simulink library "threeTethers_cl"  (R2018b)
settings: Solver=VariableStepAuto  StartTime=0.0  StopTime=10.0  RelTol=1e-3
undefined symbols (not defined in the file): grav, initEulerAngles, initPos, rho, rho_tether, rotation_sequence, sim_param, thr1Pt, thr2Pt, thr3Pt
libraries: singleTether_cl x3
settings Model: Creator=mcobb  LastModifiedBy=Erin B

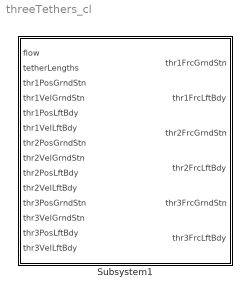
== system threeTethers_cl ==
  Subsystem1 : Subsystem

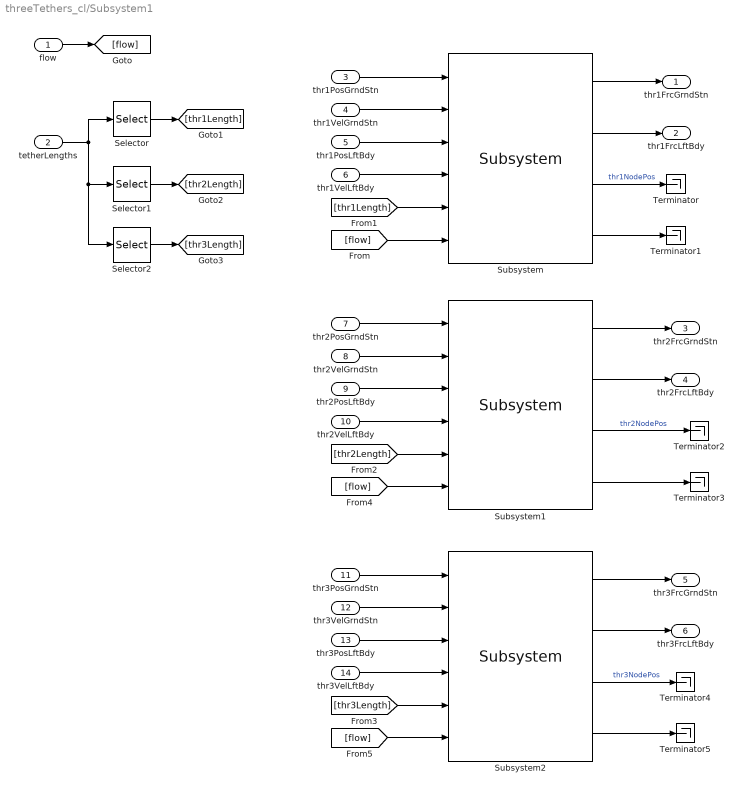
== system threeTethers_cl/Subsystem1 ==
  flow : Inport
  tetherLengths : Inport  Port=2
  thr1PosGrndStn : Inport  Port=3
  thr1VelGrndStn : Inport  Port=4
  thr1PosLftBdy : Inport  Port=5
  thr1VelLftBdy : Inport  Port=6
  thr2PosGrndStn : Inport  Port=7
  thr2VelGrndStn : Inport  Port=8
  thr2PosLftBdy : Inport  Port=9
  thr2VelLftBdy : Inport  Port=10
  thr3PosGrndStn : Inport  Port=11
  thr3VelGrndStn : Inport  Port=12
  thr3PosLftBdy : Inport  Port=13
  thr3VelLftBdy : Inport  Port=14
  Selector : Selector  InputPortWidth=3  IndexOptions=Index vector (dialog)  Indices=1  OutputSizes=1
  Selector1 : Selector  InputPortWidth=3  IndexOptions=Index vector (dialog)  Indices=2  OutputSizes=1
  Selector2 : Selector  InputPortWidth=3  IndexOptions=Index vector (dialog)  Indices=3  OutputSizes=1
  Subsystem : singleTether_cl/Subsystem  N=sim_param.N  dia_t=dia_t  E=E  rho_tether=rho + rho_tether  Cd=Cd  zeta=zeta  rho=rho  g=grav  mass=mass  ini_Rn_o=initPos + (rotation_sequence(initEulerAngles)*thr1Pt')'  ini_R1_o=thr1GndPos
  Subsystem1 : singleTether_cl/Subsystem  N=sim_param.N  dia_t=dia_t  E=E  rho_tether=rho + rho_tether  Cd=Cd  zeta=zeta  rho=rho  g=grav  mass=mass  ini_Rn_o=initPos + (rotation_sequence(initEulerAngles)*thr2Pt')'  ini_R1_o=thr2GndPos
  Subsystem2 : singleTether_cl/Subsystem  N=sim_param.N  dia_t=dia_t  E=E  rho_tether=rho + rho_tether  Cd=Cd  zeta=zeta  rho=rho  g=grav  mass=mass  ini_Rn_o=initPos + (rotation_sequence(initEulerAngles)*thr3Pt')'  ini_R1_o=thr3GndPos
  Terminator{,1..5} (6 alike) : Terminator
  thr1FrcGrndStn : Outport
  thr1FrcLftBdy : Outport  Port=2
  thr2FrcGrndStn : Outport  Port=3
  thr2FrcLftBdy : Outport  Port=4
  thr3FrcGrndStn : Outport  Port=5
  thr3FrcLftBdy : Outport  Port=6
  wires:
  thr1PosGrndStn/1 -> Subsystem/1
  thr1VelGrndStn/1 -> Subsystem/2
  thr1VelLftBdy/1 -> Subsystem/4
  thr1PosLftBdy/1 -> Subsystem/3
  flow/1 -> [flow]
  [flow] -> Subsystem/6
  Selector/1 -> [thr1Length]
  tetherLengths/1 -> Selector/1, Selector1/1, Selector2/1
  Selector1/1 -> [thr2Length]
  Selector2/1 -> [thr3Length]
  [thr1Length] -> Subsystem/5
  [thr2Length] -> Subsystem1/5
  [thr3Length] -> Subsystem2/5
  [flow] -> Subsystem1/6
  [flow] -> Subsystem2/6
  thr2PosGrndStn/1 -> Subsystem1/1
  thr2VelGrndStn/1 -> Subsystem1/2
  thr2PosLftBdy/1 -> Subsystem1/3
  thr2VelLftBdy/1 -> Subsystem1/4
  thr3VelLftBdy/1 -> Subsystem2/4
  thr3PosLftBdy/1 -> Subsystem2/3
  thr3VelGrndStn/1 -> Subsystem2/2
  thr3PosGrndStn/1 -> Subsystem2/1
  Subsystem/1 -> thr1FrcGrndStn/1
  Subsystem/2 -> thr1FrcLftBdy/1
  Subsystem/3 -> Terminator/1  "thr1NodePos"
  Subsystem/4 -> Terminator1/1
  Subsystem2/4 -> Terminator5/1
  Subsystem2/3 -> Terminator4/1  "thr3NodePos"
  Subsystem2/2 -> thr3FrcLftBdy/1
  Subsystem2/1 -> thr3FrcGrndStn/1
  Subsystem1/4 -> Terminator3/1
  Subsystem1/3 -> Terminator2/1  "thr2NodePos"
  Subsystem1/2 -> thr2FrcLftBdy/1
  Subsystem1/1 -> thr2FrcGrndStn/1
